simulink model "torque"  (R2017b)
settings: Solver=VariableStepAuto  StartTime=0.0  StopTime=10.0  RelTol=1e-3
libraries: mblibv1 x4, vrlib x1
settings Model: Creator=alinvoicu26  LastModifiedBy=alinvoicu26

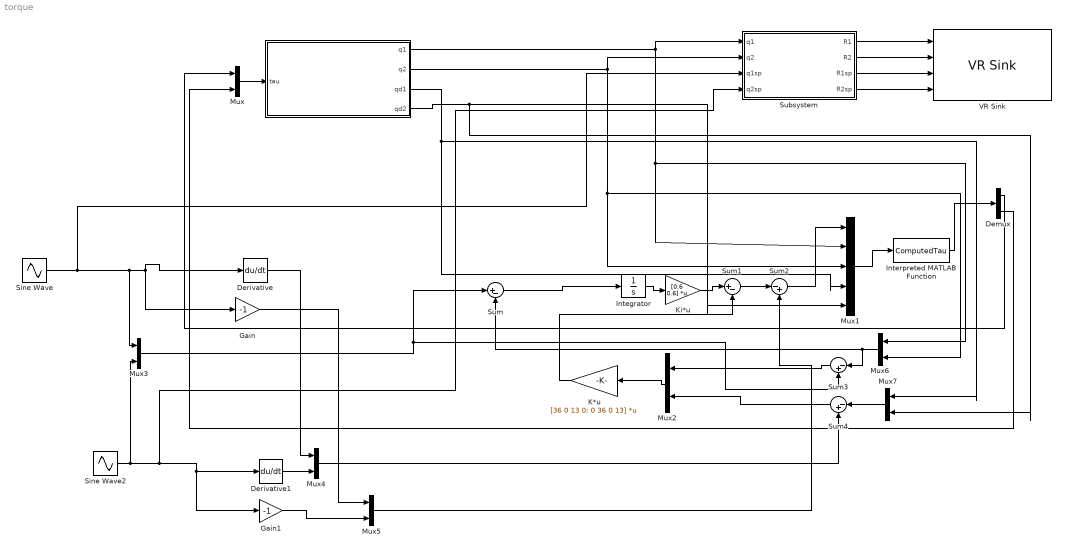
== system torque ==
  " " : Subsystem
  Demux : Demux  Outputs=2
  Derivative : Derivative
  Derivative1 : Derivative
  Gain : Gain  Gain=-1
  Gain1 : Gain  Gain=-1
  Integrator : Integrator
  Interpreted MATLAB Function : MATLABFcn  MATLABFcn=ComputedTau  OutputDimensions=2  Output1D=off
  "K*u " : Gain  Gain=[36 0 13 0; 0 36 0 13]  Multiplication=Matrix(K*u) (u vector)
  Ki*u : Gain  Gain=[0.6 0.6]  Multiplication=Matrix(K*u) (u vector)
  Mux{,2..7} (7 alike) : Mux  Inputs=2
  Mux1 : Mux  Inputs=5
  Sine Wave : Sin  SampleTime=0
  Sine Wave2 : Sin  SampleTime=0
  Subsystem : Subsystem
  Sum : Sum  Inputs=|+-
  Sum1 : Sum  Inputs=|+-
  Sum2 : Sum  Inputs=|-+
  Sum3 : Sum  Inputs=|-+
  Sum4 : Sum  Inputs=|-+
  VR Sink : vrlib/VR Sink  InstantiateOnLoad=on  SampleTime=0.1  ViewEnable=on  RemoteChange=off  RemoteView=off  FieldsWritten=Joint1.rotation.4.1.1.double#Joint2.rotation.4.1.1.double#Joint1_SP.rotation.4.1.1.double#Joint2_SP.rotation.4.1.1.double  WorldFileName=my_robot.wrl  AutoView=off  VideoDimensions=[]  AllowVariableSize=off  FigureProperties="{'Position', 'Name', 'Viewpoint', 'CameraBound', 'CameraDirection', 'CameraPosition', 'CameraUpVector', 'ZoomFactor', 'Antialiasing', 'Headlight', 'Lighting', 'NavPanel', 'Sound', 'StatusBar', 'Stereo3D', 'Stereo3DCameraOffset', 'Stereo3DHIT', 'ToolBar', 'Textures', 'Transparency', 'Triad', 'Wireframe', 'NavZones', 'NavMode', 'NavSpeed', 'CaptureFileFormat', 'CaptureFileName', 'Record2DCompressMethod', 'Record2DCompressQuality', 'Record2D', 'Record2DFileName', 'Record2DFPS'; [5.0000000000000000e+00   9.2000000000000000e+01   5.7600000000000000e+02   3.8000000000000000e+02], '', '', 'on', [0.0000000000000000e+00   0.0000000000000000e+00  -1.0000000000000000e+00], [0.0000000000000000e+00   0.0000000000000000e+00   5.1000000000000000e+01], [0.0000000000000000e+00   1.0000000000000000e+00   0.0000000000000000e+00], [1.0000000000000000e+00], 'on', 'on', 'on', 'halfbar', 'on', 'on', 'off', [1.0000000149011612e-01], [0.0000000000000000e+00], 'on', 'on', 'on', 'none', 'off', 'off', 'fly', 'normal', 'tif', '%f_anim_%n.tif', 'auto', [7.5000000000000000e+01], 'off', '%f_anim_%n.avi', 'auto'}"
      settings: SourceProductBaseCode=VR
  wires:
  Subsystem/3(R1sp) -> VR Sink/3
  " "/4(qd2) -> Mux7/2, Mux1/5
  " "/1(q1) -> Subsystem/1(q1), Mux6/1, Mux1/2
  Gain1/1 -> Mux5/2
  Ki*u/1 -> Sum1/1
  Mux2/1 -> "K*u "/1
  Sum4/1 -> Mux2/2
  Mux5/1 -> Sum2/2
  Mux4/1 -> Sum4/2
  Mux/1 -> " "/1(tau)
  Demux/2 -> Mux/2
  Sum/1 -> Integrator/1
  Demux/1 -> Mux/1
  Mux1/1 -> Interpreted MATLAB Function/1
  Gain/1 -> Mux5/1
  Mux3/1 -> Sum3/2, Sum/1
  Mux7/1 -> Sum4/1
  Mux6/1 -> Sum/2, Sum3/1
  Derivative/1 -> Mux4/1
  Interpreted MATLAB Function/1 -> Demux/1
  Subsystem/2(R2) -> VR Sink/2
  Derivative1/1 -> Mux4/2
  Sine Wave/1 -> Subsystem/3(q1sp), Mux3/1, Derivative/1, Gain/1
  " "/3(qd1) -> Mux7/1, Mux1/4
  Sine Wave2/1 -> Mux3/2, Subsystem/4(q2sp), Derivative1/1, Gain1/1
  "K*u "/1 -> Sum1/2
  Subsystem/4(R2sp) -> VR Sink/4
  Integrator/1 -> Ki*u/1
  " "/2(q2) -> Subsystem/2(q2), Mux6/2, Mux1/3
  Sum2/1 -> Mux1/1
  Subsystem/1(R1) -> VR Sink/1
  Sum1/1 -> Sum2/1
  Sum3/1 -> Mux2/1

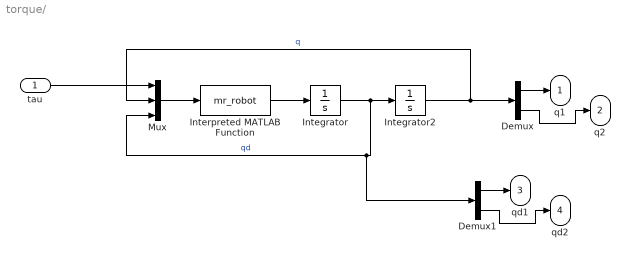
== system torque/  ==
  tau : Inport
  Demux : Demux  Outputs=2
  Demux1 : Demux  Outputs=2
  Integrator : Integrator
  Integrator2 : Integrator  InitialCondition=pi/2*0
  Interpreted MATLAB Function : MATLABFcn  MATLABFcn=mr_robot  OutputDimensions=2
  Mux : Mux  Inputs=3
  q1 : Outport
  q2 : Outport  Port=2
  qd1 : Outport  Port=3
  qd2 : Outport  Port=4
  wires:
  Interpreted MATLAB Function/1 -> Integrator/1
  Integrator2/1 -> Demux/1, Mux/2  "q"
  Integrator/1 -> Demux1/1, Mux/3, Integrator2/1  "qd"
  tau/1 -> Mux/1
  Mux/1 -> Interpreted MATLAB Function/1
  Demux/1 -> q1/1
  Demux/2 -> q2/1
  Demux1/2 -> qd2/1
  Demux1/1 -> qd1/1

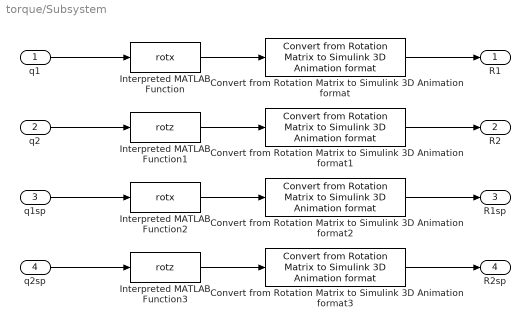
== system torque/Subsystem ==
  q1 : Inport
  q2 : Inport  Port=2
  q1sp : Inport  Port=3
  q2sp : Inport  Port=4
  Convert from Rotation Matrix to Simulink 3D Animation format{,1..3} (4 alike) : mblibv1/Utilities/Convert from Rotation Matrix to Simulink 3D Animation format
      settings: SourceProductName=Simscape Multibody  SourceProductBaseCode=MS
  Interpreted MATLAB Function : MATLABFcn  MATLABFcn=rotx
  Interpreted MATLAB Function1 : MATLABFcn  MATLABFcn=rotz
  Interpreted MATLAB Function2 : MATLABFcn  MATLABFcn=rotx
  Interpreted MATLAB Function3 : MATLABFcn  MATLABFcn=rotz
  R1 : Outport
  R2 : Outport  Port=2
  R1sp : Outport  Port=3
  R2sp : Outport  Port=4
  wires:
  Convert from Rotation Matrix to Simulink 3D Animation format/1 -> R1/1
  Interpreted MATLAB Function/1 -> Convert from Rotation Matrix to Simulink 3D Animation format/1
  Interpreted MATLAB Function1/1 -> Convert from Rotation Matrix to Simulink 3D Animation format1/1
  Interpreted MATLAB Function2/1 -> Convert from Rotation Matrix to Simulink 3D Animation format2/1
  Interpreted MATLAB Function3/1 -> Convert from Rotation Matrix to Simulink 3D Animation format3/1
  q1/1 -> Interpreted MATLAB Function/1
  q2/1 -> Interpreted MATLAB Function1/1
  q1sp/1 -> Interpreted MATLAB Function2/1
  q2sp/1 -> Interpreted MATLAB Function3/1
  Convert from Rotation Matrix to Simulink 3D Animation format1/1 -> R2/1
  Convert from Rotation Matrix to Simulink 3D Animation format2/1 -> R1sp/1
  Convert from Rotation Matrix to Simulink 3D Animation format3/1 -> R2sp/1
